simulink model "SimulationOfSystemVariableStepResponseCurve"  (Simulink 8.9)
settings: Solver=VariableStepAuto  StartTime=0.0  StopTime=10.0  RelTol=1e-3
settings Model: Creator=xiang  LastModifiedBy=xiang
settings DataIOCC: LimitDataPoints=off  SaveFormat=Dataset  SignalLoggingSaveFormat=Dataset
settings OptimizationCC: LifeSpan=auto
settings DebuggingCC: UnderspecifiedInitializationDetection=Simplified  MergeDetectMultiDrivingBlocksExec=error  FcnCallInpInsideContextMsg=error  StateNameClashWarn=none  SFUnexpectedBacktrackingDiag=error  SFNoUnconditionalDefaultTransitionDiag=error  SFExecutionAtInitializationDiag=warning
settings HardwareCC: ProdBitPerPointer=64  ProdBitPerSizeT=64  ProdBitPerPtrDiffT=64  ProdLargestAtomicFloat=Float  ProdIntDivRoundTo=Zero  ProdEndianess=LittleEndian  ProdWordSize=64  ProdHWDeviceType=Intel->x86-64 (Windows64)
settings ModelReferenceCC: PropagateSignalLabelsOutOfModel=on
settings GRTTargetCC: TargetLangStandard=C99 (ISO)  GeneratePreprocessorConditionals=Use local settings  CombineOutputUpdateFcns=on  GRTInterface=off
settings ConfigComp: CovMetricSettings=dwe  CovHtmlReporting=off  CovSaveCumulativeToWorkspaceVar=off  CovSaveSingleToWorkspaceVar=off  CovExternalEMLEnable=on

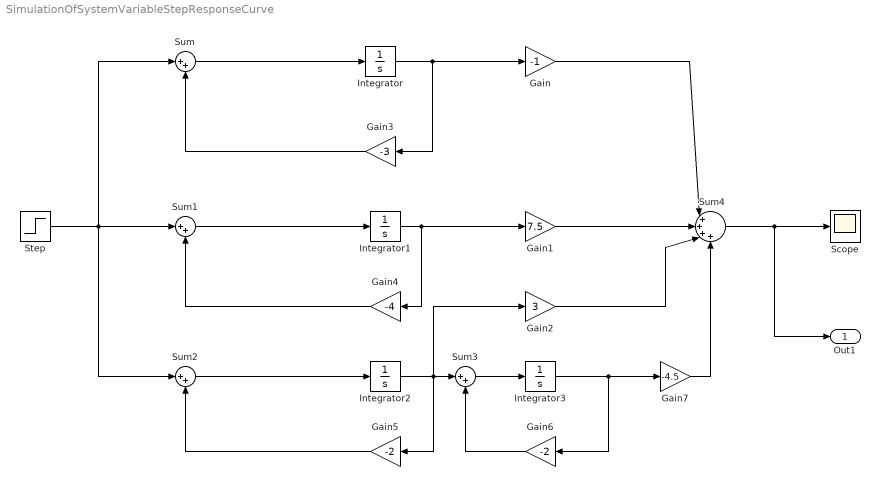
== system SimulationOfSystemVariableStepResponseCurve ==
  Gain : Gain  Gain=-1
  Gain1 : Gain  Gain=7.5
  Gain2 : Gain  Gain=3
  Gain3 : Gain  Gain=-3
  Gain4 : Gain  Gain=-4
  Gain5 : Gain  Gain=-2
  Gain6 : Gain  Gain=-2
  Gain7 : Gain  Gain=-4.5
  Integrator{,1..3} (4 alike) : Integrator
  Scope : Scope
  Step : Step  SampleTime=0
  Sum{,1..3} (4 alike) : Sum  Inputs=|++
  Sum4 : Sum  Inputs=|++++
  Out1 : Outport
  wires:
  Step/1 -> Sum2/1, Sum/1, Sum1/1
  Sum/1 -> Integrator/1
  Gain3/1 -> Sum/2
  Integrator/1 -> Gain/1, Gain3/1
  Gain/1 -> Sum4/1
  Gain1/1 -> Sum4/2
  Sum4/1 -> Out1/1, Scope/1
  Gain2/1 -> Sum4/3
  Gain7/1 -> Sum4/4
  Integrator3/1 -> Gain6/1, Gain7/1
  Integrator2/1 -> Gain5/1, Gain2/1, Sum3/1
  Sum3/1 -> Integrator3/1
  Gain6/1 -> Sum3/2
  Gain4/1 -> Sum1/2
  Sum1/1 -> Integrator1/1
  Integrator1/1 -> Gain4/1, Gain1/1
  Sum2/1 -> Integrator2/1
  Gain5/1 -> Sum2/2
